simulink model "quad_model_v4_mirko"  (R2025b)
settings: Solver=ode4  StartTime=0.0  StopTime=9  FixedStep=1/1000  RelTol=1e-6  AbsTol=1e-9
values from neighbouring files (symbols this model uses):
  p_bias = 0.7    [quad_model_v3_mirko.mat]
  P_estimated = [-0.0152071349 -2.12488163501 15.8169215204 0.213838460004 0.211325774693 0.00632668058234 -1.61230353615 8.60973613674 3.99107872735 0.549996110776 0.449999627952 0.999934525376 ... (20 elements, 20x1)]    [quad_model_v3_mirko.mat]
  q_bias = 1.4    [quad_model_v3_mirko.mat]
  r_bias = 0.3    [quad_model_v3_mirko.mat]
undefined symbols (not defined in the file or in its folder): alt, ii
libraries: matrix_library x1
settings Model: Creator=Henrique  LastModifiedBy=mirko

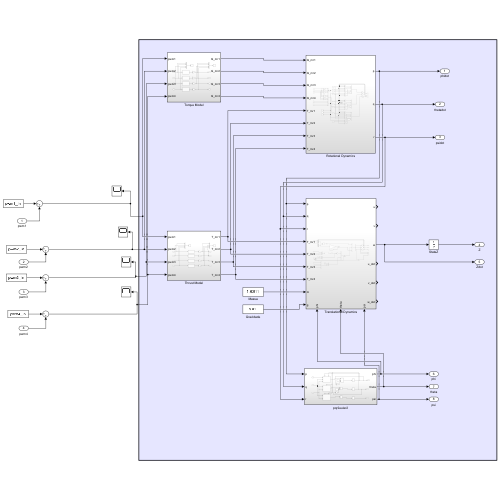
[thumbnail: Simulink's stored preview of the top-level diagram]
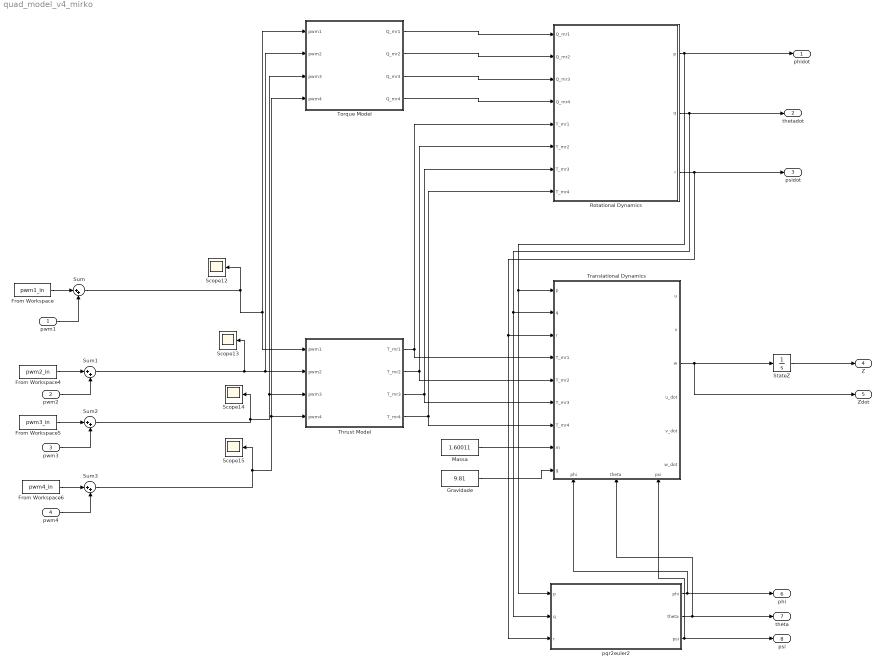
== system quad_model_v4_mirko ==
  pwm1 : Inport
  pwm2 : Inport  Port=2
  pwm3 : Inport  Port=3
  pwm4 : Inport  Port=4
  From Workspace : FromWorkspace  VariableName=pwm1_in
  From Workspace4 : FromWorkspace  VariableName=pwm2_in
  From Workspace5 : FromWorkspace  VariableName=pwm3_in
  From Workspace6 : FromWorkspace  VariableName=pwm4_in
  Gravidade : Constant  Value=9.81
  Massa : Constant  Value=1.60011
  Rotational Dynamics : Subsystem
  Scope{12..15} (4 alike) : Scope
      Scope12 settings: ActiveDisplayYMinimum=-1  ActiveDisplayYMaximum=1  DataLoggingVariableName=ScopeData16
      Scope13 settings: ActiveDisplayYMinimum=1685.1793507222485  ActiveDisplayYMaximum=1978.3134054753059  DataLoggingVariableName=ScopeData17
      Scope14 settings: ActiveDisplayYMinimum=1080.9052457228067  ActiveDisplayYMaximum=1778.9009680061222  DataLoggingVariableName=ScopeData18
      Scope15 settings: ActiveDisplayYMinimum=1275.4943161925974  ActiveDisplayYMaximum=1876.0281535711019  DataLoggingVariableName=ScopeData19
  StateZ : Integrator  InitialCondition=alt(ii)
  Sum{,1..3} (4 alike) : Sum  Inputs=|++
  Thrust Model : Subsystem
  Torque Model : Subsystem
  Translational Dynamics : Subsystem
      settings: PortSchema="{\"entries\":[{\"content\":{\"sides\":[{\"content\":{\"connectorIds\":[\"In1\",\"In2\",\"In3\",\"In4\",\"In5\",\"In6\",\"In7\",\"In8\",\"In9\"]},\"type\":\"ConnectorPlacement.EquallySpacedRectSide\",\"uuid\":\"f71b99dd-d086-42c5-ac61-061b6abdbb9c\"},{\"content\":{\"connectorIds\":[\"Out1\",\"Out2\",\"Out3\",\"Out4\",\"Out5\",\"Out6\"],\"side\":\"RIGHT\"},\"type\":\"ConnectorPlacement.EquallySpacedRectSide\",\"uuid\":\"0b5053fb-5501-424a-8925-f85dbe0224ed\"},{\"content\":{\"side\":\"TOP\"},\"type\":\"ConnectorPlacement.EquallySpacedRectSide\",\"uuid\":\"78179af8-06bb-410d-a49e-4acd134f9d12\"},{\"content\":{\"connectorIds\":[\"In10\",\"In11\",\"In12\"],\"side\":\"BOTTOM\"},\"type\":\"ConnectorPlacement.EquallySpacedRectSide\",\"uuid\":\"bdd8f061-0396-4374-a6c5-d0327680942c\"}]},\"type\":\"ConnectorPlacement.EquallySpacedConnector\",\"uuid\":\"f37cf57e-ef9d-4b35-a128-86db6ae39fb0\"}],\"packageUris\":[\"http://schema.mathworks.com/mf0/Connector/R2020b\"],\"version\":\"1.0\"}"
  pqr2euler2 : Subsystem
  phidot : Outport
  thetadot : Outport  Port=2
  psidot : Outport  Port=3
  Z : Outport  Port=4
  Zdot : Outport  Port=5
  phi : Outport  Port=6
  theta : Outport  Port=7
  psi : Outport  Port=8
  wires:
  pqr2euler2/1(phi) -> Translational Dynamics/10(phi), phi/1
  pqr2euler2/2(theta) -> Translational Dynamics/11(theta), theta/1
  Sum1/1 -> Scope13/1, Thrust Model/2(pwm2), Torque Model/2(pwm2)
  Sum2/1 -> Scope14/1, Thrust Model/3(pwm3), Torque Model/3(pwm3)
  Sum3/1 -> Scope15/1, Thrust Model/4(pwm4), Torque Model/4(pwm4)
  Thrust Model/1(T_mr1) -> Translational Dynamics/4(T_mr1), Rotational Dynamics/5(T_mr1)
  Thrust Model/2(T_mr2) -> Translational Dynamics/5(T_mr2), Rotational Dynamics/6(T_mr2)
  Thrust Model/3(T_mr3) -> Translational Dynamics/6(T_mr3), Rotational Dynamics/7(T_mr3)
  Thrust Model/4(T_mr4) -> Translational Dynamics/7(T_mr4), Rotational Dynamics/8(T_mr4)
  Massa/1 -> Translational Dynamics/8(m)
  Gravidade/1 -> Translational Dynamics/9(g)
  Sum/1 -> Thrust Model/1(pwm1), Torque Model/1(pwm1), Scope12/1
  Torque Model/1(Q_mr1) -> Rotational Dynamics/1(Q_mr1)
  Torque Model/2(Q_mr2) -> Rotational Dynamics/2(Q_mr2)
  Torque Model/3(Q_mr3) -> Rotational Dynamics/3(Q_mr3)
  Torque Model/4(Q_mr4) -> Rotational Dynamics/4(Q_mr4)
  Rotational Dynamics/3(r) -> pqr2euler2/3(r), Translational Dynamics/3(r), psidot/1
  Rotational Dynamics/1(p) -> pqr2euler2/1(p), Translational Dynamics/1(p), phidot/1
  Rotational Dynamics/2(q) -> pqr2euler2/2(q), Translational Dynamics/2(q), thetadot/1
  StateZ/1 -> Z/1
  pqr2euler2/3(psi) -> psi/1, Translational Dynamics/12(psi)
  Translational Dynamics/3(w) -> Zdot/1, StateZ/1
  pwm1/1 -> Sum/2
  From Workspace/1 -> Sum/1
  pwm2/1 -> Sum1/2
  From Workspace4/1 -> Sum1/1
  pwm3/1 -> Sum2/2
  From Workspace5/1 -> Sum2/1
  pwm4/1 -> Sum3/2
  From Workspace6/1 -> Sum3/1

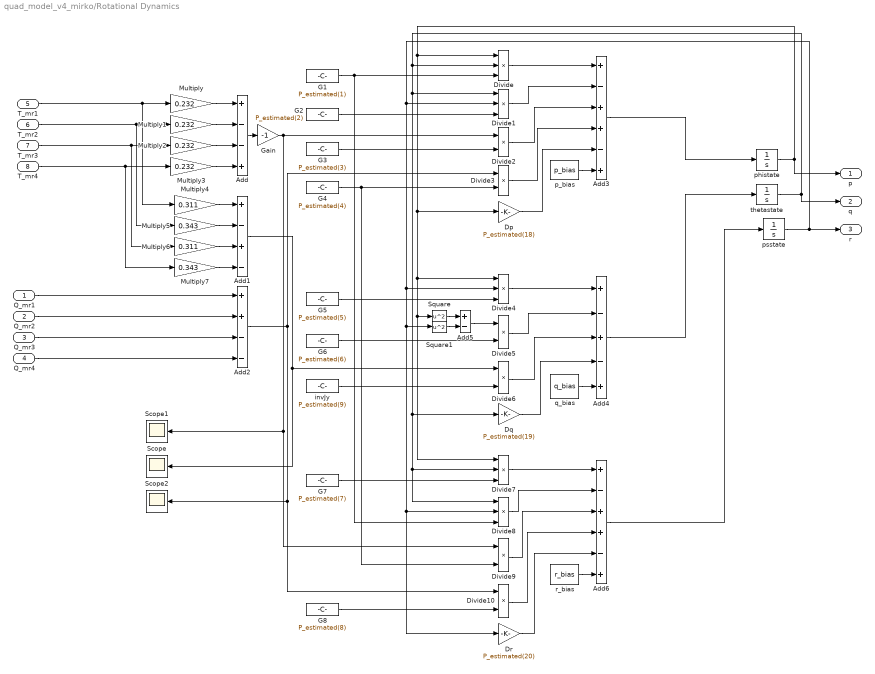
== system quad_model_v4_mirko/Rotational Dynamics ==
  Q_mr1 : Inport
  Q_mr2 : Inport  Port=2
  Q_mr3 : Inport  Port=3
  Q_mr4 : Inport  Port=4
  T_mr1 : Inport  Port=5
  T_mr2 : Inport  Port=6
  T_mr3 : Inport  Port=7
  T_mr4 : Inport  Port=8
  Add : Sum  Inputs=+--+
  Add1 : Sum  Inputs=+-+-
  Add2 : Sum  Inputs=++--
  Add3 : Sum  Inputs=+-++-+
  Add4 : Sum  Inputs=+-+-+
  Add5 : Sum  Inputs=+-
  Add6 : Sum  Inputs=+-++-+
  Divide{,1,4,7..8} (5 alike) : Product  Inputs=***
  Divide{2..3,5..6,9..10} (6 alike) : Product  Inputs=**
  Dp : Gain  Gain=P_estimated(18)
  Dq : Gain  Gain=P_estimated(19)
  Dr : Gain  Gain=P_estimated(20)
  G1 : Constant  Value=P_estimated(1)
  G2 : Constant  Value=P_estimated(2)
  G3 : Constant  Value=P_estimated(3)
  G4 : Constant  Value=P_estimated(4)
  G5 : Constant  Value=P_estimated(5)
  G6 : Constant  Value=P_estimated(6)
  G7 : Constant  Value=P_estimated(7)
  G8 : Constant  Value=P_estimated(8)
  Gain : Gain  Gain=-1
  Multiply{,1..3} (4 alike) : Gain  Gain=0.232
  Multiply4 : Gain  Gain=0.311
  Multiply5 : Gain  Gain=0.343
  Multiply6 : Gain  Gain=0.311
  Multiply7 : Gain  Gain=0.343
  Scope : Scope
      settings: ActiveDisplayYMinimum=-1.8186421464991014  ActiveDisplayYMaximum=1.3644776033104633
  Scope1 : Scope
      settings: ActiveDisplayYMinimum=-1.6294615313185898  ActiveDisplayYMaximum=1.5969792003618728  DataLoggingVariableName=ScopeData10
  Scope2 : Scope
      settings: ActiveDisplayYMinimum=-0.15040664283566432  ActiveDisplayYMaximum=0.048390422178986287  DataLoggingVariableName=ScopeData11
  Square : Math  Operator=square
  Square1 : Math  Operator=square
  invJy : Constant  Value=P_estimated(9)
  p_bias : Constant  Value=p_bias
  phistate : Integrator
  psstate : Integrator  InitialCondition=-0.1
  q_bias : Constant  Value=q_bias
  r_bias : Constant  Value=r_bias
  thetastate : Integrator  InitialCondition=-0.1
  p : Outport
  q : Outport  Port=2
  r : Outport  Port=3
  wires:
  phistate/1 -> p/1, Divide4/1, Divide7/1, Square/1, Dp/1, Divide/1
  thetastate/1 -> q/1, Divide8/1, Divide7/2, Dq/1, Divide1/1, Divide/2
  psstate/1 -> r/1, Divide4/2, Dr/1, Divide8/2, Square1/1, Divide1/2
  Multiply/1 -> Add/1
  Multiply1/1 -> Add/2
  Multiply2/1 -> Add/3
  Multiply3/1 -> Add/4
  T_mr2/1 -> Multiply5/1, Multiply1/1
  T_mr1/1 -> Multiply4/1, Multiply/1
  T_mr3/1 -> Multiply6/1, Multiply2/1
  T_mr4/1 -> Multiply7/1, Multiply3/1
  Q_mr1/1 -> Add2/1
  Q_mr2/1 -> Add2/2
  Q_mr3/1 -> Add2/3
  Q_mr4/1 -> Add2/4
  Multiply5/1 -> Add1/2
  Multiply7/1 -> Add1/4
  Multiply4/1 -> Add1/1
  Multiply6/1 -> Add1/3
  Add/1 -> Gain/1
  G1/1 -> Divide8/3, Divide/3
  G2/1 -> Divide1/3
  G3/1 -> Divide2/2
  Gain/1 -> Scope1/1, Divide9/1, Divide2/1
  G4/1 -> Divide9/2, Divide3/2
  Add2/1 -> Scope2/1, Divide10/1, Divide3/1
  Divide/1 -> Add3/1
  Divide1/1 -> Add3/2
  Divide2/1 -> Add3/3
  Divide3/1 -> Add3/4
  Dp/1 -> Add3/5
  p_bias/1 -> Add3/6
  Add3/1 -> phistate/1
  G5/1 -> Divide4/3
  Square/1 -> Add5/1
  Square1/1 -> Add5/2
  Divide4/1 -> Add4/1
  Add5/1 -> Divide5/1
  G6/1 -> Divide5/2
  invJy/1 -> Divide6/2
  Add1/1 -> Scope/1, Divide6/1
  Divide5/1 -> Add4/2
  Divide6/1 -> Add4/3
  Dq/1 -> Add4/4
  q_bias/1 -> Add4/5
  Add4/1 -> thetastate/1
  Divide7/1 -> Add6/1
  G7/1 -> Divide7/3
  Divide8/1 -> Add6/2
  G8/1 -> Divide10/2
  Divide9/1 -> Add6/3
  Divide10/1 -> Add6/4
  r_bias/1 -> Add6/6
  Dr/1 -> Add6/5
  Add6/1 -> psstate/1

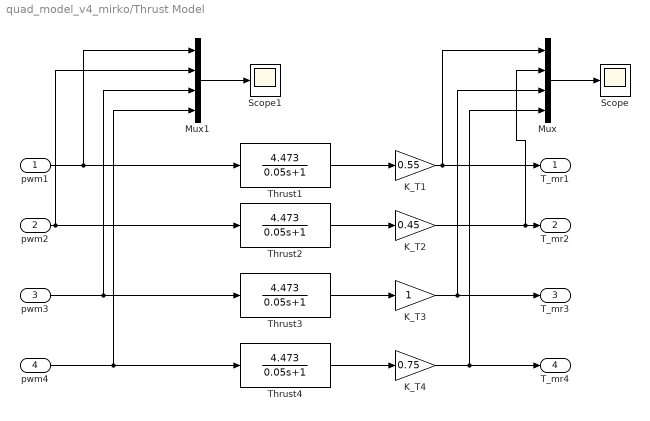
== system quad_model_v4_mirko/Thrust Model ==
  pwm1 : Inport
  pwm2 : Inport  Port=2
  pwm3 : Inport  Port=3
  pwm4 : Inport  Port=4
  K_T1 : Gain  Gain=0.55
  K_T2 : Gain  Gain=0.45
  K_T3 : Gain
  K_T4 : Gain  Gain=0.75
  Mux : Mux
  Mux1 : Mux
  Scope : Scope
      settings: ActiveDisplayYMinimum=-942.12961691203509  ActiveDisplayYMaximum=8479.1665522083185
  Scope1 : Scope
      settings: ActiveDisplayYMinimum=1050.1250000000364  ActiveDisplayYMaximum=2048.8749999999959
  Thrust{1..4} (4 alike) : TransferFcn  Numerator=4.473  Denominator=[0.05 1]
  T_mr1 : Outport
  T_mr2 : Outport  Port=2
  T_mr3 : Outport  Port=3
  T_mr4 : Outport  Port=4
  wires:
  Mux/1 -> Scope/1
  Mux1/1 -> Scope1/1
  pwm2/1 -> Thrust2/1, Mux1/2
  pwm3/1 -> Thrust3/1, Mux1/3
  pwm1/1 -> Thrust1/1, Mux1/1
  pwm4/1 -> Thrust4/1, Mux1/4
  K_T1/1 -> Mux/1, T_mr1/1
  K_T2/1 -> Mux/2, T_mr2/1
  K_T3/1 -> Mux/3, T_mr3/1
  K_T4/1 -> Mux/4, T_mr4/1
  Thrust1/1 -> K_T1/1
  Thrust2/1 -> K_T2/1
  Thrust3/1 -> K_T3/1
  Thrust4/1 -> K_T4/1

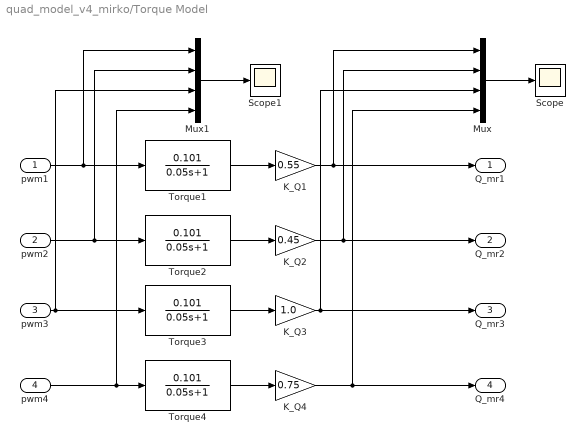
== system quad_model_v4_mirko/Torque Model ==
  pwm1 : Inport
  pwm2 : Inport  Port=2
  pwm3 : Inport  Port=3
  pwm4 : Inport  Port=4
  K_Q1 : Gain  Gain=0.55
  K_Q2 : Gain  Gain=0.45
  K_Q3 : Gain  Gain=1.0
  K_Q4 : Gain  Gain=0.75
  Mux : Mux
  Mux1 : Mux
  Scope : Scope
      settings: ActiveDisplayYMinimum=-21.273215137070324  ActiveDisplayYMaximum=191.45893623363295
  Scope1 : Scope
      settings: ActiveDisplayYMinimum=620.06953512003383  ActiveDisplayYMaximum=2620.0695351200338
  Torque{1..4} (4 alike) : TransferFcn  Numerator=0.101  Denominator=[0.05 1]
  Q_mr1 : Outport
  Q_mr2 : Outport  Port=2
  Q_mr3 : Outport  Port=3
  Q_mr4 : Outport  Port=4
  wires:
  Mux/1 -> Scope/1
  Mux1/1 -> Scope1/1
  pwm2/1 -> Torque2/1, Mux1/2
  pwm3/1 -> Torque3/1, Mux1/3
  pwm1/1 -> Torque1/1, Mux1/1
  pwm4/1 -> Torque4/1, Mux1/4
  Torque4/1 -> K_Q4/1
  Torque3/1 -> K_Q3/1
  Torque2/1 -> K_Q2/1
  Torque1/1 -> K_Q1/1
  K_Q1/1 -> Mux/1, Q_mr1/1
  K_Q2/1 -> Mux/2, Q_mr2/1
  K_Q3/1 -> Mux/3, Q_mr3/1
  K_Q4/1 -> Q_mr4/1, Mux/4

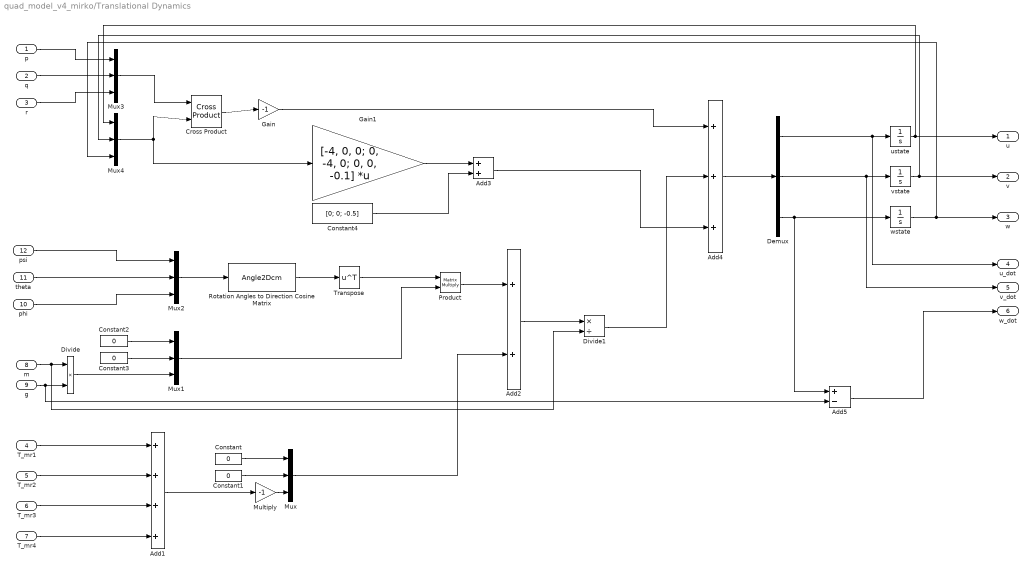
== system quad_model_v4_mirko/Translational Dynamics ==
  p : Inport
  q : Inport  Port=2
  r : Inport  Port=3
  T_mr1 : Inport  Port=4
  T_mr2 : Inport  Port=5
  T_mr3 : Inport  Port=6
  T_mr4 : Inport  Port=7
  m : Inport  Port=8
  g : Inport  Port=9
  phi : Inport  Port=10
  theta : Inport  Port=11
  psi : Inport  Port=12
  Add1 : Sum  Inputs=++++
  Add2 : Sum
  Add3 : Sum
  Add4 : Sum  Inputs=+++
  Add5 : Sum  Inputs=+-
  Constant{,1..3} (4 alike) : Constant  Value=0
  Constant4 : Constant  Value=[0; 0; -0.5]
  Cross Product : matrix_library/Cross Product
  Demux : Demux  Outputs=3
  Divide : Product  Inputs=**
  Divide1 : Product  Inputs=*/
  Gain : Gain  Gain=-1
  Gain1 : Gain  Gain=[-4, 0, 0; 0, -4, 0; 0, 0, -0.1]  Multiplication=Matrix(K*u)
  Multiply : Gain  Gain=-1
  Mux{,1..4} (5 alike) : Mux  Inputs=3
  Product : Product  Multiplication=Matrix(*)
  Rotation Angles to Direction Cosine Matrix : Angle2Dcm
      settings: AttributesFormatString=Rotation Order: %<rotationOrder>
  Transpose : Math  Operator=transpose
  ustate : Integrator
  vstate : Integrator
  wstate : Integrator
  u : Outport
  v : Outport  Port=2
  w : Outport  Port=3
  u_dot : Outport  Port=4
  v_dot : Outport  Port=5
  w_dot : Outport  Port=6
  wires:
  Multiply/1 -> Mux/3
  Add1/1 -> Multiply/1
  Constant/1 -> Mux/1
  Constant1/1 -> Mux/2
  T_mr4/1 -> Add1/4
  T_mr3/1 -> Add1/3
  T_mr2/1 -> Add1/2
  T_mr1/1 -> Add1/1
  Constant3/1 -> Mux1/2
  Constant2/1 -> Mux1/1
  Divide/1 -> Mux1/3
  m/1 -> Divide1/2, Divide/1
  g/1 -> Add5/2, Divide/2
  psi/1 -> Mux2/1
  theta/1 -> Mux2/2
  phi/1 -> Mux2/3
  Mux2/1 -> Rotation Angles to Direction Cosine Matrix/1
  Rotation Angles to Direction Cosine Matrix/1 -> Transpose/1
  Transpose/1 -> Product/1
  Mux1/1 -> Product/2
  Product/1 -> Add2/1
  Mux/1 -> Add2/2
  p/1 -> Mux3/1
  q/1 -> Mux3/2
  r/1 -> Mux3/3
  Mux3/1 -> Cross Product/1
  Mux4/1 -> Gain1/1, Cross Product/2
  Cross Product/1 -> Gain/1
  Add2/1 -> Divide1/1
  Gain1/1 -> Add3/1
  Constant4/1 -> Add3/2
  Gain/1 -> Add4/1
  Divide1/1 -> Add4/2
  Add3/1 -> Add4/3
  Add4/1 -> Demux/1
  Demux/2 -> v_dot/1, vstate/1
  Demux/3 -> Add5/1, wstate/1
  Demux/1 -> u_dot/1, ustate/1
  ustate/1 -> u/1, Mux4/1
  vstate/1 -> Mux4/2, v/1
  wstate/1 -> Mux4/3, w/1
  Add5/1 -> w_dot/1

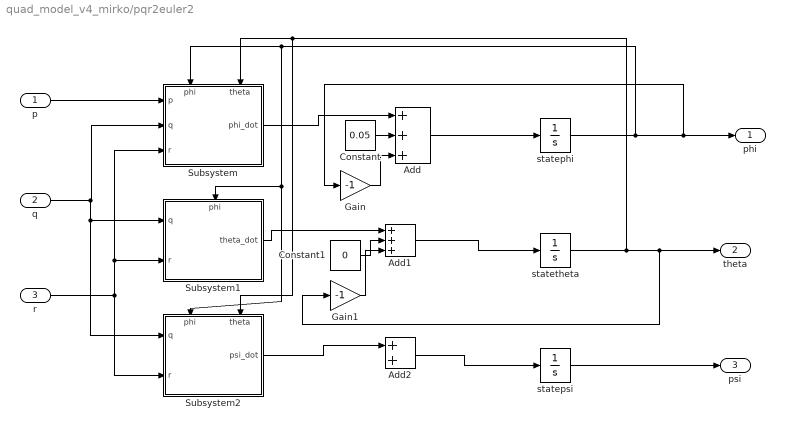
== system quad_model_v4_mirko/pqr2euler2 ==
  p : Inport
  q : Inport  Port=2
  r : Inport  Port=3
  Add : Sum  Inputs=+++
  Add1 : Sum  Inputs=+++
  Add2 : Sum
  Constant : Constant  Value=0.05
  Constant1 : Constant  Value=0
  Gain : Gain  Gain=-1
  Gain1 : Gain  Gain=-1
  Subsystem : Subsystem
      settings: PortSchema="{\"entries\":[{\"content\":{\"sides\":[{\"content\":{\"connectorIds\":[\"In1\",\"In2\",\"In3\"]},\"type\":\"ConnectorPlacement.EquallySpacedRectSide\",\"uuid\":\"382c9118-e079-49d8-ab8c-004ad07464e7\"},{\"content\":{\"connectorIds\":[\"Out1\"],\"side\":\"RIGHT\"},\"type\":\"ConnectorPlacement.EquallySpacedRectSide\",\"uuid\":\"72894542-f6bc-4d77-962a-2bf0bb014da1\"},{\"content\":{\"connectorIds\":[\"In4\",\"In5\"],\"side\":\"TOP\"},\"type\":\"ConnectorPlacement.EquallySpacedRectSide\",\"uuid\":\"7c36585a-f7f1-487a-9d1f-f469af8d2b77\"}]},\"type\":\"ConnectorPlacement.EquallySpacedConnector\",\"uuid\":\"a2cbdec5-7730-4b32-9373-0b6b5d68d7f2\"}],\"packageUris\":[\"http://schema.mathworks.com/mf0/Connector/R2020b\"],\"version\":\"1.0\"}"
  Subsystem1 : Subsystem
      settings: PortSchema="{\"entries\":[{\"content\":{\"sides\":[{\"content\":{\"connectorIds\":[\"In1\",\"In2\"]},\"type\":\"ConnectorPlacement.EquallySpacedRectSide\",\"uuid\":\"382c9118-e079-49d8-ab8c-004ad07464e7\"},{\"content\":{\"connectorIds\":[\"Out1\"],\"side\":\"RIGHT\"},\"type\":\"ConnectorPlacement.EquallySpacedRectSide\",\"uuid\":\"72894542-f6bc-4d77-962a-2bf0bb014da1\"},{\"content\":{\"connectorIds\":[\"In3\"],\"side\":\"TOP\"},\"type\":\"ConnectorPlacement.EquallySpacedRectSide\",\"uuid\":\"7c36585a-f7f1-487a-9d1f-f469af8d2b77\"}]},\"type\":\"ConnectorPlacement.EquallySpacedConnector\",\"uuid\":\"a2cbdec5-7730-4b32-9373-0b6b5d68d7f2\"}],\"packageUris\":[\"http://schema.mathworks.com/mf0/Connector/R2020b\"],\"version\":\"1.0\"}"
  Subsystem2 : Subsystem
      settings: PortSchema="{\"entries\":[{\"content\":{\"sides\":[{\"content\":{\"connectorIds\":[\"In1\",\"In2\"]},\"type\":\"ConnectorPlacement.EquallySpacedRectSide\",\"uuid\":\"382c9118-e079-49d8-ab8c-004ad07464e7\"},{\"content\":{\"connectorIds\":[\"Out1\"],\"side\":\"RIGHT\"},\"type\":\"ConnectorPlacement.EquallySpacedRectSide\",\"uuid\":\"72894542-f6bc-4d77-962a-2bf0bb014da1\"},{\"content\":{\"connectorIds\":[\"In3\",\"In4\"],\"side\":\"TOP\"},\"type\":\"ConnectorPlacement.EquallySpacedRectSide\",\"uuid\":\"7c36585a-f7f1-487a-9d1f-f469af8d2b77\"}]},\"type\":\"ConnectorPlacement.EquallySpacedConnector\",\"uuid\":\"a2cbdec5-7730-4b32-9373-0b6b5d68d7f2\"}],\"packageUris\":[\"http://schema.mathworks.com/mf0/Connector/R2020b\"],\"version\":\"1.0\"}"
  statephi : Integrator  InitialCondition=-0.0291
  statepsi : Integrator  InitialCondition=3.3486
  statetheta : Integrator  InitialCondition=0.0103
  phi : Outport
  theta : Outport  Port=2
  psi : Outport  Port=3
  wires:
  statephi/1 -> Subsystem2/3(phi), Subsystem1/3(phi), Subsystem/4(phi), Gain/1, phi/1
  statetheta/1 -> Subsystem2/4(theta), Subsystem/5(theta), Gain1/1, theta/1
  statepsi/1 -> psi/1
  p/1 -> Subsystem/1(p)
  q/1 -> Subsystem2/1(q), Subsystem1/1(q), Subsystem/2(q)
  r/1 -> Subsystem2/2(r), Subsystem1/2(r), Subsystem/3(r)
  Subsystem/1(phi_dot) -> Add/1
  Add/1 -> statephi/1
  Add1/1 -> statetheta/1
  Subsystem1/1(theta_dot) -> Add1/1
  Add2/1 -> statepsi/1
  Subsystem2/1(psi_dot) -> Add2/1
  Constant/1 -> Add/2
  Constant1/1 -> Add1/2
  Gain/1 -> Add/3
  Gain1/1 -> Add1/3

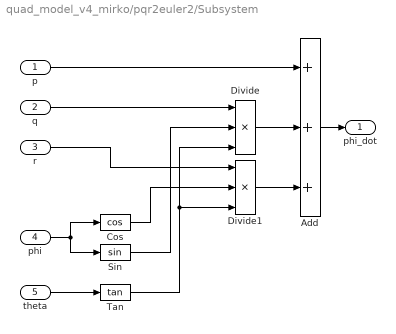
== system quad_model_v4_mirko/pqr2euler2/Subsystem ==
  p : Inport
  q : Inport  Port=2
  r : Inport  Port=3
  phi : Inport  Port=4
  theta : Inport  Port=5
  Add : Sum  Inputs=+++
  Cos : Trigonometry  Operator=cos
  Divide : Product  Inputs=***
  Divide1 : Product  Inputs=***
  Sin : Trigonometry
  Tan : Trigonometry  Operator=tan
  phi_dot : Outport
  wires:
  Add/1 -> phi_dot/1
  Divide1/1 -> Add/3
  Divide/1 -> Add/2
  p/1 -> Add/1
  phi/1 -> Sin/1, Cos/1
  theta/1 -> Tan/1
  q/1 -> Divide/1
  Sin/1 -> Divide/2
  Tan/1 -> Divide1/3, Divide/3
  r/1 -> Divide1/1
  Cos/1 -> Divide1/2

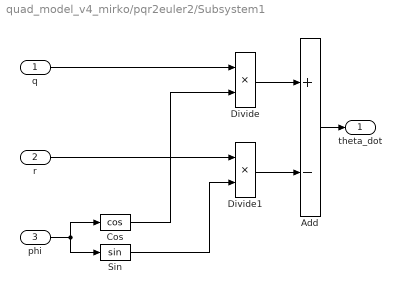
== system quad_model_v4_mirko/pqr2euler2/Subsystem1 ==
  q : Inport
  r : Inport  Port=2
  phi : Inport  Port=3
  Add : Sum  Inputs=+-
  Cos : Trigonometry  Operator=cos
  Divide : Product  Inputs=**
  Divide1 : Product  Inputs=**
  Sin : Trigonometry
  theta_dot : Outport
  wires:
  Add/1 -> theta_dot/1
  phi/1 -> Sin/1, Cos/1
  q/1 -> Divide/1
  r/1 -> Divide1/1
  Cos/1 -> Divide/2
  Sin/1 -> Divide1/2
  Divide/1 -> Add/1
  Divide1/1 -> Add/2

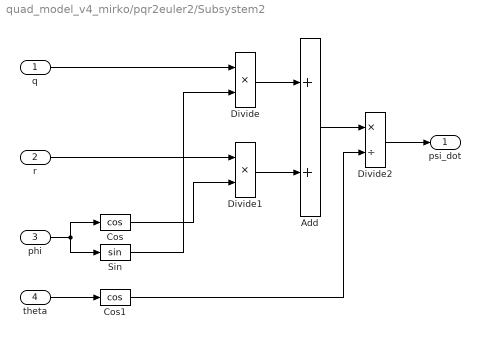
== system quad_model_v4_mirko/pqr2euler2/Subsystem2 ==
  q : Inport
  r : Inport  Port=2
  phi : Inport  Port=3
  theta : Inport  Port=4
  Add : Sum
  Cos : Trigonometry  Operator=cos
  Cos1 : Trigonometry  Operator=cos
  Divide : Product  Inputs=**
  Divide1 : Product  Inputs=**
  Divide2 : Product  Inputs=*/
  Sin : Trigonometry
  psi_dot : Outport
  wires:
  phi/1 -> Sin/1, Cos/1
  Divide/1 -> Add/1
  Divide1/1 -> Add/2
  theta/1 -> Cos1/1
  Add/1 -> Divide2/1
  Cos1/1 -> Divide2/2
  q/1 -> Divide/1
  Sin/1 -> Divide/2
  r/1 -> Divide1/1
  Cos/1 -> Divide1/2
  Divide2/1 -> psi_dot/1
